simulink model "Non_lin_template_2015a"  (R2015a)
settings: Solver=ode45  SolverMode=SingleTasking  StartTime=0.0  StopTime=10.0  RelTol=1e-3
undefined symbols (not defined in the file or in its folder): delta_f, delta_r, v_des
libraries: simulink x1
settings Model: CovMetricSettings=dwe  CovHtmlReporting=off  covSaveCumulativeToWorkspaceVar=off  CovSaveSingleToWorkspaceVar=off  CovExternalEMLEnable=on  Creator=Instructor  LastModifiedBy=Santo
settings DataIOCC: LimitDataPoints=off  SaveFormat=Dataset
settings DebuggingCC: SFUnexpectedBacktrackingDiag=error  SFNoUnconditionalDefaultTransitionDiag=error
settings HardwareCC: ProdBitPerPointer=64  ProdLargestAtomicFloat=Float  ProdIntDivRoundTo=Zero  ProdEndianess=LittleEndian  ProdHWDeviceType=Specified
settings ModelReferenceCC: PropagateSignalLabelsOutOfModel=on
settings GRTTargetCC: TargetLangStandard=C99 (ISO)  GeneratePreprocessorConditionals=Use local settings

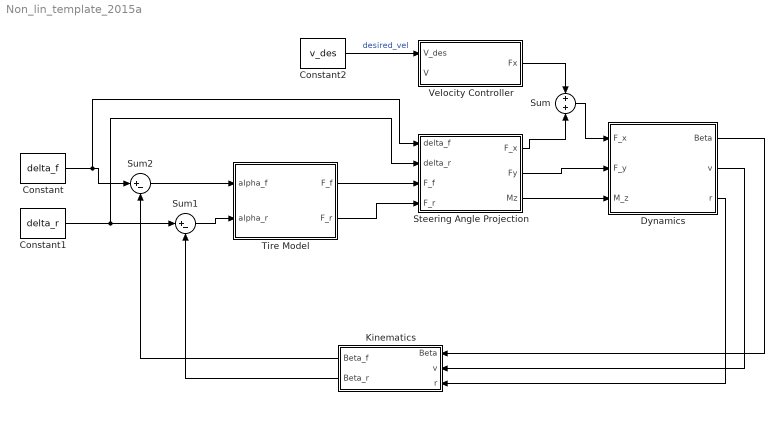
== system Non_lin_template_2015a ==
  Constant : Constant  Value=delta_f
  Constant1 : Constant  Value=delta_r
  Constant2 : Constant  Value=v_des
  Dynamics : Subsystem
  Kinematics : Subsystem
  Steering Angle Projection : Subsystem
  Sum : Sum
  Sum1 : Sum  Inputs=|+-
  Sum2 : Sum  Inputs=|+-
  Tire Model : Subsystem
  Velocity Controller : Subsystem
  wires:
  Dynamics/1(Beta) -> Kinematics/1(Beta)
  Dynamics/2(v) -> Kinematics/2(v)
  Dynamics/3(r) -> Kinematics/3(r)
  Tire Model/1(F_f) -> Steering Angle Projection/3(F_f)
  Tire Model/2(F_r) -> Steering Angle Projection/4(F_r)
  Steering Angle Projection/2(Fy) -> Dynamics/2(F_y)
  Steering Angle Projection/1(F_x) -> Sum/2
  Steering Angle Projection/3(Mz) -> Dynamics/3(M_z)
  Sum2/1 -> Tire Model/1(alpha_f)
  Sum1/1 -> Tire Model/2(alpha_r)
  Kinematics/2(Beta_r) -> Sum1/2
  Constant1/1 -> Steering Angle Projection/2(delta_r), Sum1/1
  Constant/1 -> Steering Angle Projection/1(delta_f), Sum2/1
  Kinematics/1(Beta_f) -> Sum2/2
  Velocity Controller/1(Fx) -> Sum/1
  Sum/1 -> Dynamics/1(F_x)
  Constant2/1 -> Velocity Controller/1(V_des)  "desired_vel"

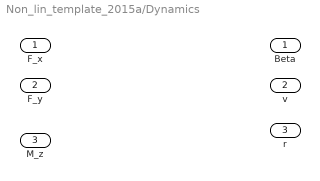
== system Non_lin_template_2015a/Dynamics ==
  F_x : Inport
  F_y : Inport  Port=2
  M_z : Inport  Port=3
  Beta : Outport
  v : Outport  Port=2
  r : Outport  Port=3

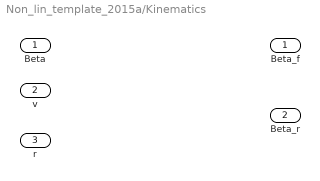
== system Non_lin_template_2015a/Kinematics ==
  Beta : Inport
  v : Inport  Port=2
  r : Inport  Port=3
  Beta_f : Outport
  Beta_r : Outport  Port=2

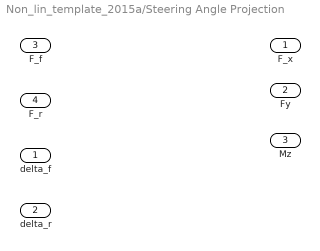
== system Non_lin_template_2015a/Steering Angle Projection ==
  delta_f : Inport
  delta_r : Inport  Port=2
  F_f : Inport  Port=3
  F_r : Inport  Port=4
  F_x : Outport
  Fy : Outport  Port=2
  Mz : Outport  Port=3

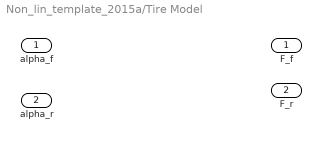
== system Non_lin_template_2015a/Tire Model ==
  alpha_f : Inport
  alpha_r : Inport  Port=2
  F_f : Outport
  F_r : Outport  Port=2

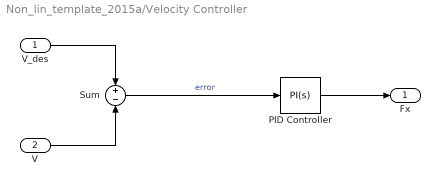
== system Non_lin_template_2015a/Velocity Controller ==
  V_des : Inport
  V : Inport  Port=2
  PID Controller : simulink/Continuous/PID Controller  Controller=PI  TimeDomain=Continuous-time  SampleTime=-1  IntegratorMethod=Forward Euler  FilterMethod=Forward Euler  Form=Parallel  UseFilter=on  ControllerParametersSource=internal  P=1  I=1  D=0  N=100  InitialConditionSource=internal  InitialConditionForIntegrator=0  InitialConditionForFilter=0  ExternalReset=none  LimitOutput=off  UpperSaturationLimit=inf  LowerSaturationLimit=-inf  LinearizeAsGain=on  AntiWindupMode=none  Kb=1  TrackingMode=off  Kt=1  PParamMin=[]  PParamMax=[]  IParamMin=[]  IParamMax=[]  DParamMin=[]  DParamMax=[]  NParamMin=[]  NParamMax=[]  KbParamMin=[]  KbParamMax=[]  KtParamMin=[]  KtParamMax=[]  POutMin=[]  POutMax=[]  IOutMin=[]  IOutMax=[]  DOutMin=[]  DOutMax=[]  NOutMin=[]  NOutMax=[]  KbOutMin=[]  KbOutMax=[]  KtOutMin=[]  KtOutMax=[]  IntegratorOutMin=[]  IntegratorOutMax=[]  FilterOutMin=[]  FilterOutMax=[]  SumOutMin=[]  SumOutMax=[]  SumI1OutMin=[]  SumI1OutMax=[]  SumI2OutMin=[]  SumI2OutMax=[]  SumI3OutMin=[]  SumI3OutMax=[]  SumDOutMin=[]  SumDOutMax=[]  SaturationOutMin=[]  SaturationOutMax=[]  IntegratorContinuousStateAttributes=''  IntegratorStateMustResolveToSignalObject=off  IntegratorRTWStateStorageClass=Auto  FilterContinuousStateAttributes=''  FilterStateMustResolveToSignalObject=off  FilterRTWStateStorageClass=Auto  DifferentiatorICPrevScaledInput=0  DifferentiatorOutMin=[]  DifferentiatorOutMax=[]
  Sum : Sum  Inputs=+-
  Fx : Outport
  wires:
  PID Controller/1 -> Fx/1
  V_des/1 -> Sum/1
  V/1 -> Sum/2
  Sum/1 -> PID Controller/1  "error"
